simulink model "PID_HeadlessTrackingControllerVariableQuadDynamicsMdl"  (R2016b)
settings: Solver=FixedStepAuto  StartTime=0.0  StopTime=30  FixedStep=0.1  RelTol=1e-3  EnableMultiTasking=on
undefined symbols (not defined in the file): Params, QuaternionController_nav, TrackingWaypoint
settings Model: Creator=Raj  LastModifiedBy=sailingpc
settings DataIOCC: LimitDataPoints=on  SaveFormat=Array
settings OptimizationCC: LifeSpan=inf
settings DebuggingCC: UnderspecifiedInitializationDetection=Classic  MergeDetectMultiDrivingBlocksExec=none  SolverPrmCheckMsg=warning  StateNameClashWarn=warning  SFUnexpectedBacktrackingDiag=warning  SFNoUnconditionalDefaultTransitionDiag=warning  SFExecutionAtInitializationDiag=none
settings HardwareCC: ProdBitPerPointer=32  ProdBitPerSizeT=32  ProdBitPerPtrDiffT=32  ProdLargestAtomicFloat=None  ProdIntDivRoundTo=Undefined  ProdEndianess=Unspecified  ProdWordSize=32  ProdHWDeviceType=32-bit Generic
settings ModelReferenceCC: PropagateSignalLabelsOutOfModel=off
settings GRTTargetCC: TargetLangStandard=C89/C90 (ANSI)  GeneratePreprocessorConditionals=Disable all
settings ConfigComp: CovMetricSettings=dw  CovHtmlReporting=on  CovSaveCumulativeToWorkspaceVar=on  CovSaveSingleToWorkspaceVar=on  CovExternalEMLEnable=off  CovSFcnEnable=off

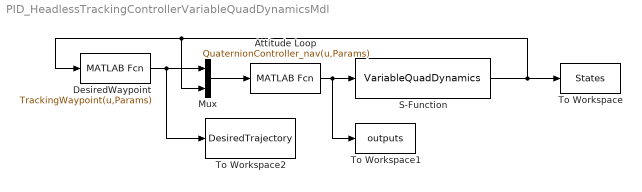
== system PID_HeadlessTrackingControllerVariableQuadDynamicsMdl ==
  Attitude Loop : MATLABFcn  MATLABFcn=QuaternionController_nav(u,Params)  OutputDimensions=4
  DesiredWaypoint : MATLABFcn  MATLABFcn=TrackingWaypoint(u,Params)  OutputDimensions=4
  Mux : Mux  Inputs=2
  S-Function : S-Function  FunctionName=VariableQuadDynamics  Parameters=Params  SFunctionDeploymentMode=off  EnableBusSupport=off
  To Workspace : ToWorkspace  VariableName=States  SaveFormat=Timeseries  SampleTime=-1
  To Workspace1 : ToWorkspace  VariableName=outputs  SaveFormat=Timeseries  SampleTime=-1
  To Workspace2 : ToWorkspace  VariableName=DesiredTrajectory  SaveFormat=Timeseries  SampleTime=-1
  wires:
  Attitude Loop/1 -> S-Function/1, To Workspace1/1
  Mux/1 -> Attitude Loop/1
  DesiredWaypoint/1 -> Mux/1, To Workspace2/1
  S-Function/1 -> DesiredWaypoint/1, Mux/2, To Workspace/1
